simulink model "Analisis_Respuesta_Temporal_Simulink"  (R2014a)
settings: Solver=ode45  StartTime=0.0  StopTime=40  RelTol=1e-3
values from neighbouring files (symbols this model uses):
  k = 1    [Analisis_Respuesta_Temporal.m]    (also in Analisis_Respuesta_Temporal_segundo_orden.m; Masa_Resorte_Duro_Parametros.m = 0.5; Representacion_en_Espacio_Estados.m)
  tao1 = -1    [Analisis_Respuesta_Temporal.m]
  tao2 = 5    [Analisis_Respuesta_Temporal.m]
  tao3 = 0.2    [Analisis_Respuesta_Temporal.m]
settings Model: Creator=Jose  LastModifiedBy=Jose

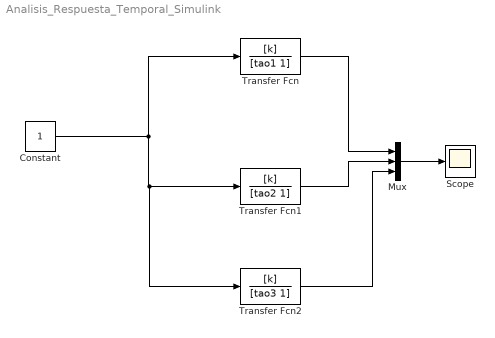
== system Analisis_Respuesta_Temporal_Simulink ==
  Constant : Constant
  Mux : Mux  Inputs=3
  Scope : Scope
  Transfer Fcn : TransferFcn  Numerator=[k]  Denominator=[tao1 1]
  Transfer Fcn1 : TransferFcn  Numerator=[k]  Denominator=[tao2 1]
  Transfer Fcn2 : TransferFcn  Numerator=[k]  Denominator=[tao3 1]
  wires:
  Constant/1 -> Transfer Fcn/1, Transfer Fcn2/1, Transfer Fcn1/1
  Transfer Fcn/1 -> Mux/1
  Transfer Fcn1/1 -> Mux/2
  Transfer Fcn2/1 -> Mux/3
  Mux/1 -> Scope/1
